simulink model "structuri_avansate_de_control"  (R2022b)
settings: Solver=FixedStepAuto  StartTime=0.0  StopTime=900  FixedStep=0.01  RelTol=1e-3
values from neighbouring files (symbols this model uses):
  C = 5.6    [CalculeProiect.m]
  h0 = 13.97    [CalculeProiect.m]
  h1 = 17.85    [CalculeProiect.m]
  k = 0.024    [CalculeProiect.m]
  k1 = 0.624    [CalculeProiect.m]
  k11 = k2*k2+4*(k-k3)*k1    (= 0.0616266)    [CalculeProiect.m]
  k12 = 8*(k-k3)    (= 0.1968)    [CalculeProiect.m]
  k13 = 2*(k-k3)    (= 0.0492)    [CalculeProiect.m]
  k2 = -0.015    [CalculeProiect.m]
  k3 = -0.0006    [CalculeProiect.m]
  kcompensare = (delta_h/(q1-q0))/(delta_h/delta_ua)    (= 0.185185185185)    [CalculeProiect.m]
  kp = (delta_h/3)/delta_ua    (= 2.58666666667)    [CalculeProiect.m]
  q0 = 20.97    [CalculeProiect.m]
undefined symbols (not defined in the file or in its folder): ki, ki1, ki2, kp1, kp2
libraries: slpidlib x6
(part 2 of 2)

== system structuri_avansate_de_control/ModelProces 3/Pompa/k12 ==
  k : Inport
  Product1 : Product
  Subtract : Sum  Inputs=+-
  "constant " : Constant  Value=8
  k3 : Constant  Value=k3
  k12 : Outport
  wires:
  k/1 -> Subtract/1
  k3/1 -> Subtract/2
  Subtract/1 -> Product1/1
  "constant "/1 -> Product1/2
  Product1/1 -> k12/1

== system structuri_avansate_de_control/ModelProces 3/Pompa/k13 ==
  k : Inport
  Product1 : Product
  Subtract : Sum  Inputs=+-
  "constant " : Constant  Value=2
  k3 : Constant  Value=k3
  k13 : Outport
  wires:
  k/1 -> Subtract/1
  k3/1 -> Subtract/2
  Subtract/1 -> Product1/1
  "constant "/1 -> Product1/2
  Product1/1 -> k13/1

== system structuri_avansate_de_control/cascada/Pompa/k11  ==
  k : Inport
  Add : Sum
  Constant : Constant  Value=4
  Product : Product
  Product1 : Product  Inputs=3
  Subtract : Sum  Inputs=+-
  k1 : Constant  Value=k1
  k2 : Constant  Value=k2
  k3 : Constant  Value=k3
  k11 : Outport
  wires:
  k2/1 -> Product/2, Product/1
  k/1 -> Subtract/1
  k3/1 -> Subtract/2
  Subtract/1 -> Product1/1
  k1/1 -> Product1/2
  Constant/1 -> Product1/3
  Product1/1 -> Add/1
  Product/1 -> Add/2
  Add/1 -> k11/1

== system structuri_avansate_de_control/cascada/Pompa/k12 ==
  k : Inport
  Product1 : Product
  Subtract : Sum  Inputs=+-
  "constant " : Constant  Value=8
  k3 : Constant  Value=k3
  k12 : Outport
  wires:
  k/1 -> Subtract/1
  k3/1 -> Subtract/2
  Subtract/1 -> Product1/1
  "constant "/1 -> Product1/2
  Product1/1 -> k12/1

== system structuri_avansate_de_control/cascada/Pompa/k13 ==
  k : Inport
  Product1 : Product
  Subtract : Sum  Inputs=+-
  "constant " : Constant  Value=2
  k3 : Constant  Value=k3
  k13 : Outport
  wires:
  k/1 -> Subtract/1
  k3/1 -> Subtract/2
  Subtract/1 -> Product1/1
  "constant "/1 -> Product1/2
  Product1/1 -> k13/1

== system structuri_avansate_de_control/perturbatie intrare + iesire/Pompa/k11  ==
  k : Inport
  Add : Sum
  Constant : Constant  Value=4
  Product : Product
  Product1 : Product  Inputs=3
  Subtract : Sum  Inputs=+-
  k1 : Constant  Value=k1
  k2 : Constant  Value=k2
  k3 : Constant  Value=k3
  k11 : Outport
  wires:
  k2/1 -> Product/2, Product/1
  k/1 -> Subtract/1
  k3/1 -> Subtract/2
  Subtract/1 -> Product1/1
  k1/1 -> Product1/2
  Constant/1 -> Product1/3
  Product1/1 -> Add/1
  Product/1 -> Add/2
  Add/1 -> k11/1

== system structuri_avansate_de_control/perturbatie intrare + iesire/Pompa/k12 ==
  k : Inport
  Product1 : Product
  Subtract : Sum  Inputs=+-
  "constant " : Constant  Value=8
  k3 : Constant  Value=k3
  k12 : Outport
  wires:
  k/1 -> Subtract/1
  k3/1 -> Subtract/2
  Subtract/1 -> Product1/1
  "constant "/1 -> Product1/2
  Product1/1 -> k12/1

== system structuri_avansate_de_control/perturbatie intrare + iesire/Pompa/k13 ==
  k : Inport
  Product1 : Product
  Subtract : Sum  Inputs=+-
  "constant " : Constant  Value=2
  k3 : Constant  Value=k3
  k13 : Outport
  wires:
  k/1 -> Subtract/1
  k3/1 -> Subtract/2
  Subtract/1 -> Product1/1
  "constant "/1 -> Product1/2
  Product1/1 -> k13/1
